simulink model "dinamica"  (Simulink 8.8)
settings: Solver=VariableStepAuto  StartTime=0.0  StopTime=tempo_simulacao  RelTol=1e-3  EnableMultiTasking=on
libraries: roblocks x3, simulink x1
settings Model: Creator=arthu  LastModifiedBy=juan
settings SolverCC: MaxOrder=2  MaxConsecutiveMinStep=50
settings DataIOCC: LimitDataPoints=off  SaveFormat=Dataset  SignalLoggingSaveFormat=Dataset
settings DebuggingCC: UnderspecifiedInitializationDetection=Simplified  MergeDetectMultiDrivingBlocksExec=error  FcnCallInpInsideContextMsg=error  StateNameClashWarn=none
settings HardwareCC: ProdBitPerPointer=64  ProdBitPerSizeT=64  ProdBitPerPtrDiffT=64  ProdLargestAtomicFloat=Float  ProdIntDivRoundTo=Zero  ProdEndianess=LittleEndian  ProdWordSize=64  ProdHWDeviceType=Intel->x86-64 (Windows64)
settings ModelReferenceCC: PropagateSignalLabelsOutOfModel=on
settings GRTTargetCC: CombineOutputUpdateFcns=on  GRTInterface=off

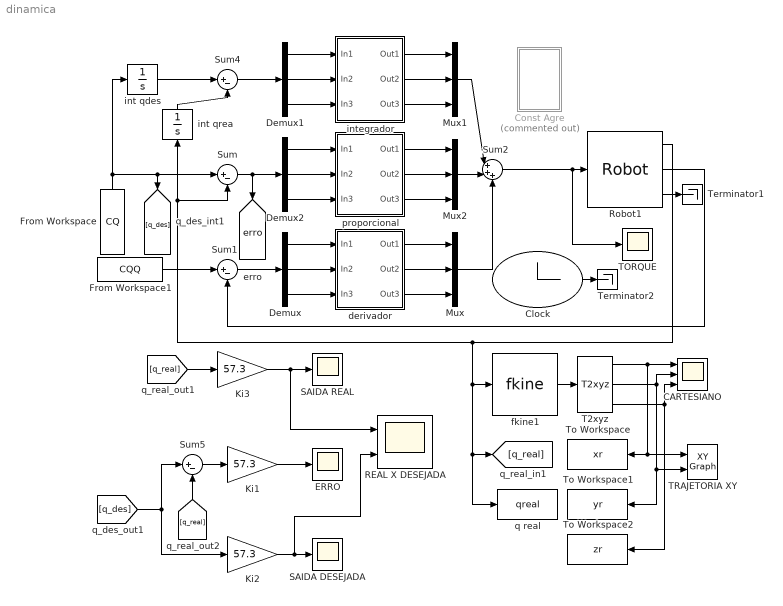
== system dinamica ==
  CARTESIANO : Scope  NumInputPorts=3
  Clock : Clock
  Const Agre : Subsystem  Commented=on
  Demux : Demux  Outputs=3
  Demux1 : Demux  Outputs=3
  Demux2 : Demux  Outputs=3
  ERRO : Scope
  From Workspace : FromWorkspace  VariableName=CQ  SampleTime=0
  From Workspace1 : FromWorkspace  VariableName=CQQ  SampleTime=0
  Ki1 : Gain  Gain=57.3  SaturateOnIntegerOverflow=on  OutDataTypeStr=Inherit: Same as input  ParamDataTypeStr=Inherit: Same as input
  Ki2 : Gain  Gain=57.3  SaturateOnIntegerOverflow=on  OutDataTypeStr=Inherit: Same as input  ParamDataTypeStr=Inherit: Same as input
  Ki3 : Gain  Gain=57.3  SaturateOnIntegerOverflow=on  OutDataTypeStr=Inherit: Same as input  ParamDataTypeStr=Inherit: Same as input
  Mux : Mux  Inputs=3
  Mux1 : Mux  Inputs=3
  Mux2 : Mux  Inputs=3
  REAL X DESEJADA : Scope  NumInputPorts=2
  Robot1 : roblocks/Arm/Robot  robot=robot  q0=[0 0 0]
  SAIDA DESEJADA : Scope
  SAIDA REAL : Scope
  Sum{,1,4..5} (4 alike) : Sum  Inputs=|+-  SaturateOnIntegerOverflow=on  InputSameDT=on  OutDataTypeStr=Inherit: Same as first input
  Sum2 : Sum  Inputs=|+++  SaturateOnIntegerOverflow=on  InputSameDT=on  OutDataTypeStr=Inherit: Same as first input
  T2xyz : roblocks/Toolbox/T2xyz
  TORQUE : Scope
  TRAJETORIA XY : simulink/Sinks/XY Graph  xmin=0  xmax=0.23  ymin=-0.23  ymax=0.23  st=-1
  Terminator1 : Terminator
  Terminator2 : Terminator
  To Workspace : ToWorkspace  VariableName=xr  SampleTime=-1
  To Workspace1 : ToWorkspace  VariableName=yr  SampleTime=-1
  To Workspace2 : ToWorkspace  VariableName=zr  SampleTime=-1
  derivador : Subsystem
  fkine1 : roblocks/Arm/fkine  robot=robot
  int qdes : Integrator
  int qrea : Integrator
  integrador : Subsystem
  proporcional : Subsystem
  q real : ToWorkspace  VariableName=qreal  SampleTime=-1
  tag scope: erro=global
  wires:
  Robot1/1 -> int qrea/1, Sum/2, fkine1/1, [q_real], q real/1
  Robot1/3 -> Terminator1/1
  Clock/1 -> Terminator2/1
  From Workspace1/1 -> Sum1/1
  Ki2/1 -> REAL X DESEJADA/2, SAIDA DESEJADA/1
  int qrea/1 -> Sum4/2
  int qdes/1 -> Sum4/1
  Robot1/2 -> Sum1/2
  Ki1/1 -> ERRO/1
  Sum5/1 -> Ki1/1
  Sum1/1 -> Demux/1
  Demux/1 -> derivador/1(In1)
  Demux/2 -> derivador/2(In2)
  Demux/3 -> derivador/3(In3)
  derivador/1(Out1) -> Mux/1
  derivador/2(Out2) -> Mux/2
  derivador/3(Out3) -> Mux/3
  Mux/1 -> Sum2/3
  Demux1/2 -> integrador/2(In2)
  integrador/2(Out2) -> Mux1/2
  integrador/1(Out1) -> Mux1/1
  integrador/3(Out3) -> Mux1/3
  Demux1/1 -> integrador/1(In1)
  Demux1/3 -> integrador/3(In3)
  Sum4/1 -> Demux1/1
  Mux1/1 -> Sum2/1
  proporcional/2(Out2) -> Mux2/2
  proporcional/1(Out1) -> Mux2/1
  proporcional/3(Out3) -> Mux2/3
  Demux2/1 -> proporcional/1(In1)
  Demux2/2 -> proporcional/2(In2)
  Sum/1 -> Demux2/1, [erro]
  Demux2/3 -> proporcional/3(In3)
  Mux2/1 -> Sum2/2
  fkine1/1 -> T2xyz/1
  T2xyz/1 -> CARTESIANO/1, TRAJETORIA XY/1, To Workspace/1
  T2xyz/2 -> CARTESIANO/2, To Workspace1/1, TRAJETORIA XY/2
  T2xyz/3 -> CARTESIANO/3, To Workspace2/1
  From Workspace/1 -> [q_des], Sum/1, int qdes/1
  [q_des] -> Sum5/1, Ki2/1
  [q_real] -> Sum5/2
  Ki3/1 -> REAL X DESEJADA/1, SAIDA REAL/1
  [q_real] -> Ki3/1
  Sum2/1 -> TORQUE/1, Robot1/1

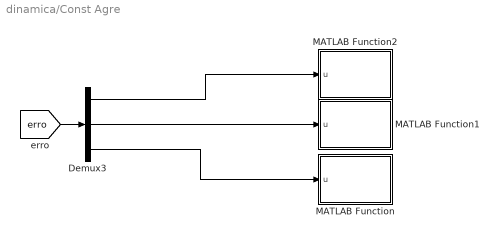
== system dinamica/Const Agre ==
  Demux3 : Demux  Outputs=3
  MATLAB Function : MATLAB Function  TreatAsAtomicUnit=on
  MATLAB Function1 : MATLAB Function  TreatAsAtomicUnit=on
  MATLAB Function2 : MATLAB Function  TreatAsAtomicUnit=on
  wires:
  [erro] -> Demux3/1
  Demux3/3 -> MATLAB Function/1(u)
  Demux3/2 -> MATLAB Function1/1(u)
  Demux3/1 -> MATLAB Function2/1(u)

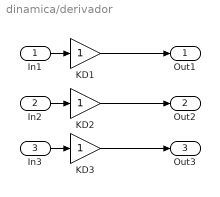
== system dinamica/derivador ==
  In1 : Inport
  In2 : Inport  Port=2
  In3 : Inport  Port=3
  KD1 : Gain
  KD2 : Gain
  KD3 : Gain
  Out1 : Outport
  Out2 : Outport  Port=2
  Out3 : Outport  Port=3
  wires:
  In3/1 -> KD3/1
  KD3/1 -> Out3/1
  KD1/1 -> Out1/1
  KD2/1 -> Out2/1
  In1/1 -> KD1/1
  In2/1 -> KD2/1

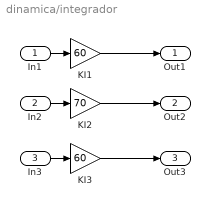
== system dinamica/integrador ==
  In1 : Inport
  In2 : Inport  Port=2
  In3 : Inport  Port=3
  KI1 : Gain  Gain=60
  KI2 : Gain  Gain=70
  KI3 : Gain  Gain=60
  Out1 : Outport
  Out2 : Outport  Port=2
  Out3 : Outport  Port=3
  wires:
  KI3/1 -> Out3/1
  KI2/1 -> Out2/1
  In2/1 -> KI2/1
  In3/1 -> KI3/1
  In1/1 -> KI1/1
  KI1/1 -> Out1/1

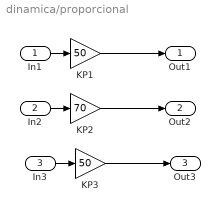
== system dinamica/proporcional ==
  In1 : Inport
  In2 : Inport  Port=2
  In3 : Inport  Port=3
  KP1 : Gain  Gain=50
  KP2 : Gain  Gain=70
  KP3 : Gain  Gain=50
  Out1 : Outport
  Out2 : Outport  Port=2
  Out3 : Outport  Port=3
  wires:
  In3/1 -> KP3/1
  KP1/1 -> Out1/1
  In1/1 -> KP1/1
  KP2/1 -> Out2/1
  In2/1 -> KP2/1
  KP3/1 -> Out3/1

== matlab function Const Agre/MATLAB Function1 ==
  data: u input double
function fcn(u)
coder.extrinsic('set_param');
if(u<0.2)
    set_param('dinamica/proporcional/KP2','Gain','50');
    set_param('dinamica/integrador/KI2','Gain','60');
    set_param('dinamica/derivador/KD2','Gain','2');
else
    set_param('dinamica/proporcional/KP2','Gain','5');
    set_param('dinamica/integrador/KI2','Gain','2');
    set_param('dinamica/derivador/KD2','Gain','1');
end
end

== matlab function Const Agre/MATLAB Function ==
  data: u input double
function fcn(u)
coder.extrinsic('set_param');
if(u<0.2)
    set_param('dinamica/proporcional/KP3','Gain','50');
    set_param('dinamica/integrador/KI3','Gain','60');
    set_param('dinamica/derivador/KD3','Gain','2');
else
    set_param('dinamica/proporcional/KP3','Gain','5');
    set_param('dinamica/integrador/KI3','Gain','2');
    set_param('dinamica/derivador/KD3','Gain','1');
end
end

== matlab function Const Agre/MATLAB Function2 ==
  data: u input double
function fcn(u)
coder.extrinsic('set_param');
if(u<0.2)
    set_param('dinamica/proporcional/KP1','Gain','50');
    set_param('dinamica/integrador/KI1','Gain','60');
    set_param('dinamica/derivador/KD1','Gain','2');
else
    set_param('dinamica/proporcional/KP1','Gain','5');
    set_param('dinamica/integrador/KI1','Gain','2');
    set_param('dinamica/derivador/KD1','Gain','1');
end
end
